simulink model "Two_DOF_Robot_v01"  (R2024b)
settings: Solver=ode45  StartTime=0.0  StopTime=10  FixedStep=Ts  RelTol=1e-3
settings Model: Creator=ababaei  LastModifiedBy=ababaei
settings SolverCC: AlgebraicLoopSolver=LineSearch
settings DataIOCC: ExternalInput=[spg.setpoint.t, dist.Fz_IH]
settings DebuggingCC: AlgebraicLoopMsg=error  ArtificialAlgebraicLoopMsg=none  UnconnectedInputMsg=warning  UnconnectedOutputMsg=warning  UnconnectedLineMsg=warning  UnderSpecifiedDimensionMsg=warning  ArithmeticOperatorsInVariantConditions=warning
settings ModelReferenceCC: EnableRefExpFcnMdlSchedulingChecks=on
settings SFSimCC: SimUseLocalCustomCode=off  CustomCodeUndefinedFunction=UseInterfaceOnly
settings RTWCC: RTWUseLocalCustomCode=off  GPUComputeCapability=3.5
settings CodeAppCC: StateflowObjectComments=on

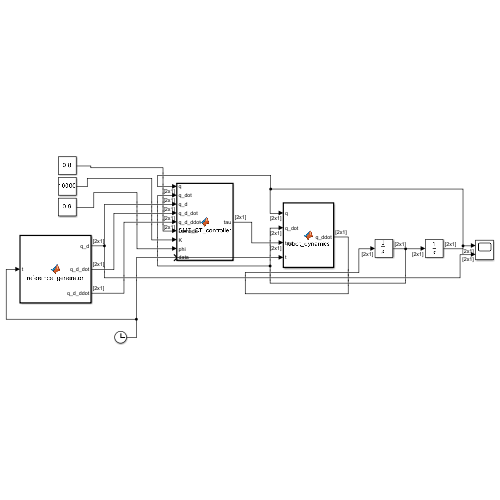
[thumbnail: Simulink's stored preview of the top-level diagram]
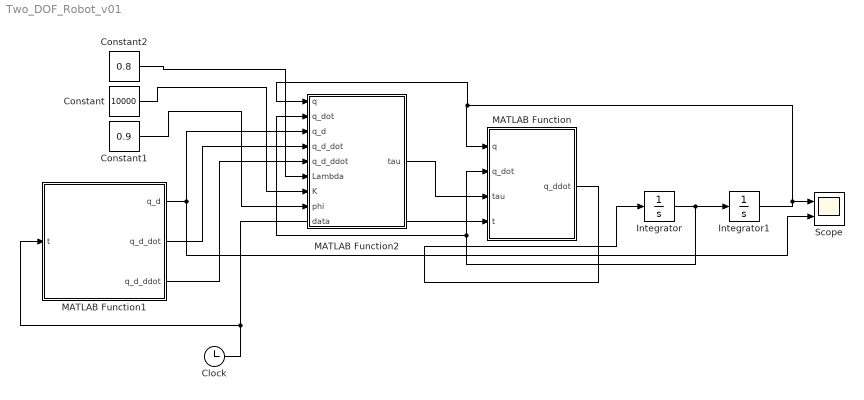
== system Two_DOF_Robot_v01 ==
  Clock : Clock
  Constant : Constant  Value=10000
  Constant1 : Constant  Value=0.9
  Constant2 : Constant  Value=0.8
  Integrator : Integrator
  Integrator1 : Integrator
  MATLAB Function : MATLAB Function  TreatAsAtomicUnit=on
  MATLAB Function1 : MATLAB Function  TreatAsAtomicUnit=on
  MATLAB Function2 : MATLAB Function  TreatAsAtomicUnit=on
  Scope : Scope  NumInputPorts=2
  wires:
  Clock/1 -> MATLAB Function/4(t), MATLAB Function1/1(t)
  MATLAB Function/1(q_ddot) -> Integrator/1
  Integrator1/1 -> MATLAB Function2/1(q), MATLAB Function/1(q), Scope/1
  Integrator/1 -> MATLAB Function/2(q_dot), MATLAB Function2/2(q_dot), Integrator1/1
  MATLAB Function2/1(tau) -> MATLAB Function/3(tau)
  MATLAB Function1/2(q_d_dot) -> MATLAB Function2/4(q_d_dot)
  MATLAB Function1/3(q_d_ddot) -> MATLAB Function2/5(q_d_ddot)
  Constant1/1 -> MATLAB Function2/8(phi)
  Constant/1 -> MATLAB Function2/7(K)
  Constant2/1 -> MATLAB Function2/6(Lambda)
  MATLAB Function1/1(q_d) -> MATLAB Function2/3(q_d), Scope/2

== matlab function Two_DOF_Robot_v01/MATLAB Function1 ==
  data: q_d output; t input; q_d_dot output; q_d_ddot output
% Below is original 
% function [q_d, q_d_dot, q_d_ddot] = reference_trajectory(t)
% % Input: time t
% % Outputs: desired position, velocity, acceleration (2×1 each)
% 
% % Joint 1 desired trajectory
% q1_d = 0.5*sin(0.5*t);
% q1_d_dot = 0.25*cos(0.5*t);          % derivative: 0.5*0.5*cos(0.5t)
% q1_d_ddot = -0.125*sin(0.5*t);       % second derivative
% 
% % Joint 2 desired trajectory  
% q2_d = 0.3*sin(0.8*t + pi/4);
% q2_d_dot = 0.24*cos(0.8*t + pi/4);   % derivative: 0.3*0.8*cos(...)
% q2_d_ddot = -0.192*sin(0.8*t + pi/4); % second derivative
% 
% q_d = [q1_d; q2_d];
% q_d_dot = [q1_d_dot; q2_d_dot];
% q_d_ddot = [q1_d_ddot; q2_d_ddot];
% end
% Below is revised input / reference signal 
function [q_d, q_d_dot, q_d_ddot] = reference_generator(t)
% Input: time t (scalar)
% Outputs: desired position, velocity, acceleration (all 2×1 vectors)

q1_d = 0.5*sin(0.5*t);                    % Joint 1 desired angle
q1_d_dot = 0.25*cos(0.5*t);               % Joint 1 desired velocity
q1_d_ddot = -0.125*sin(0.5*t);            % Joint 1 desired acceleration

q2_d = 0.3*sin(0.8*t + pi/4);             % Joint 2 desired angle
q2_d_dot = 0.24*cos(0.8*t + pi/4);        % Joint 2 desired velocity
q2_d_ddot = -0.192*sin(0.8*t + pi/4);     % Joint 2 desired acceleration

q_d = [q1_d; q2_d];                       % 2×1 position vector
q_d_dot = [q1_d_dot; q2_d_dot];           % 2×1 velocity vector
q_d_ddot = [q1_d_ddot; q2_d_ddot];        % 2×1 acceleration vector
end

== matlab function Two_DOF_Robot_v01/MATLAB Function ==
  data: q input; q_ddot output; q_dot input; tau input; t input
function q_ddot = robot_dynamics(q, q_dot, tau, t)
% Inputs:
%   q, q_dot: joint positions/velocities (2×1)
%   tau: control torque (2×1)
%   t: time (scalar)
% Output: q_ddot (2×1 acceleration)

% Robot parameters
m1=2; m2=1; l1=1; l2=1; lc1=0.5; lc2=0.5; I1=0.2; I2=0.1; g=9.81;

% Extract states
q1=q(1); q2=q(2); q1dot=q_dot(1); q2dot=q_dot(2);

% Dynamics matrices
c2=cos(q2); s2=sin(q2); c12=cos(q1+q2);

M11 = I1+I2+m1*lc1^2+m2*(l1^2+lc2^2+2*l1*lc2*c2);
M12 = I2+m2*(lc2^2+l1*lc2*c2);
M21 = M12;
M22 = I2+m2*lc2^2;
M = [M11,M12; M21,M22];

h = m2*l1*lc2*s2;
C11 = -h*q2dot;
C12 = -h*(q1dot+q2dot);
C21 = h*q1dot;
C22 = 0;
C = [C11,C12; C21,C22];

G1 = (m1*lc1+m2*l1)*g*cos(q1) + m2*lc2*g*c12;
G2 = m2*lc2*g*c12;
G = [G1; G2];

% Time-varying payload disturbance
mp = 0.5 + 0.3*sin(0.5*pi*t);            % Payload mass
F_ext = [0; -mp*g];                       % External force

% Jacobian
J = [-l1*sin(q1)-l2*sin(q1+q2), -l2*sin(q1+q2);
      l1*cos(q1)+l2*cos(q1+q2),  l2*cos(q1+q2)];
tau_disturbance = J' * F_ext;             % Disturbance torque

% Total acceleration
q_ddot = M \ (tau + tau_disturbance - C*q_dot - G);
end

== matlab function Two_DOF_Robot_v01/MATLAB Function2 ==
  data: q input; tau output size=[2 1]; q_dot input size=[2 1]; q_d input; q_d_dot input; q_d_ddot input; Lambda input; K input; phi input; data input
function tau = SMC_CT_controller(q, q_dot, q_d, q_d_dot, q_d_ddot, Lambda, K, phi, data)
% Model-based (computed-torque) sliding mode

% dynamics matrices (same as in robot_dynamics)
m1=2; m2=1; l1=1; l2=1; lc1=0.5; lc2=0.5; I1=0.2; I2=0.1; g=9.81;
q1=q(1); q2=q(2); q1dot=q_dot(1); q2dot=q_dot(2);
c2=cos(q2); s2=sin(q2); c12=cos(q1+q2);

M11 = I1+I2+m1*lc1^2+m2*(l1^2+lc2^2+2*l1*lc2*c2);
M12 = I2+m2*(lc2^2+l1*lc2*c2);
M22 = I2+m2*lc2^2;
M = [M11 M12; M12 M22];

h = m2*l1*lc2*s2;
C = [-h*q2dot, -h*(q1dot+q2dot);
      h*q1dot,  0];

G = [(m1*lc1+m2*l1)*g*cos(q1) + m2*lc2*g*c12;
      m2*lc2*g*c12];

% errors
e    = q_d - q;
e_dot= q_d_dot - q_dot;
s    = e_dot + Lambda.*e;

phi  = max(phi, 1e-6);
sat  = min(max(s./phi, -1), 1);

% 
% force 2×1 column vectors (and phi 2×1)
% q       = reshape(q,      2,1);
% q_dot   = reshape(q_dot,  2,1);
% q_d     = reshape(q_d,    2,1);
% q_d_dot = reshape(q_d_dot,2,1);
% q_d_ddot= reshape(q_d_ddot,2,1);
% 
% Lambda  = reshape(Lambda, 2,1);
% K       = reshape(K,      2,1);
% phi     = reshape(phi,    2,1);

% tau     = zeros(2,1);   % keep this too

%
% computed-torque + robust term
tau = zeros(2, 1);
tau = M*(q_d_ddot + Lambda.*e_dot) + C*q_dot + G + K.*sat;
end
